simulink model "SIR_test"  (R2018b)
settings: Solver=VariableStepAuto  StartTime=0.0  StopTime=120  RelTol=1e-3
settings Model: Creator=emcoates  LastModifiedBy=emcoates

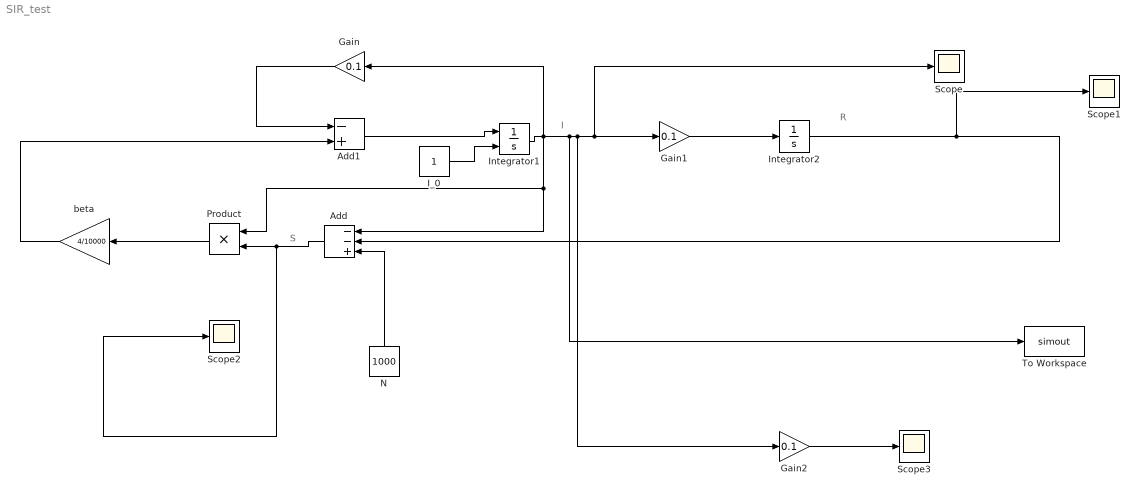
== system SIR_test ==
  note: R
  note: I
  note: S
  Add : Sum  Inputs=--+
  Add1 : Sum  Inputs=-+
  Gain : Gain  Gain=0.1
  Gain1 : Gain  Gain=0.1
  Gain2 : Gain  Gain=0.1
  I_0 : Constant
  Integrator1 : Integrator  InitialConditionSource=external
  Integrator2 : Integrator
  N : Constant  Value=1000
  Product : Product
  Scope{,1..3} (4 alike) : Scope
  To Workspace : ToWorkspace  VariableName=simout  SaveFormat=Timeseries  SampleTime=-1
  beta : Gain  Gain=4/10000
  wires:
  N/1 -> Add/3
  Integrator2/1 -> Scope1/1, Add/2
  Integrator1/1 -> To Workspace/1, Gain2/1, Scope/1, Gain1/1, Product/1, Add/1, Gain/1
  Product/1 -> beta/1
  Add/1 -> Scope2/1, Product/2
  beta/1 -> Add1/2
  Gain/1 -> Add1/1
  Add1/1 -> Integrator1/1
  Gain1/1 -> Integrator2/1
  I_0/1 -> Integrator1/2
  Gain2/1 -> Scope3/1
